simulink model "ATRIAS_vnmc"  (R2015a)
settings: Solver=ode45  StartTime=0.0  StopTime=60  FixedStep=1e-3  MinStep=1e-6  RelTol=1e-3  AbsTol=1e-4
values from neighbouring files (symbols this model uses):
  initial_boom_yaw = initial_boom_yaw + delta_yaw0    [run_model.m]
  max_floor_diff = cost_fun_opts.max_floor_diff    [opt_cmaes.m]    (also in run_model.m; set_all_params_simple.m = 0)
  noise_on_off = cost_fun_opts.noise_on_off    [opt_cmaes.m]    (also in run_model.m; set_all_params_simple.m = 0)
  noise_seed = cost_fun_opts.noise_seed    [opt_cmaes.m]    (also in run_model.m; set_all_params_simple.m = 1)
  noise_variance = cost_fun_opts.noise_variance    [opt_cmaes.m]    (also in run_model.m; set_all_params_simple.m = 0.000174532925199)
  SEA_swing_ctrl_on_off = cost_fun_opts.SEA_swing_ctrl_on_off    [opt_cmaes.m]    (also in run_model.m; set_all_params_simple.m = 0)
  sim_t = simout.twalk    [run_model.m]
  steady_dist = cost_fun_opts.steady_dist    [opt_cmaes.m]    (also in run_model.m; set_all_params_simple.m = 10)
  ts_anim = 0.0333    [run_model.m]
undefined symbols (not defined in the file or in its folder): A1_notch_f1, A2_notch_f1, A_lpf_dtau, A_lpf_velocity, B1_lpf_dtau, B1_lpf_velocity, B1_notch_f1, B2_lpf_dtau, B2_lpf_velocity, B2_notch_f1, b_hmotor, b_leg_spring, b_rotor, base_color_d, boom_color_d, boom_mount_to_center_diagonal, breakaway_friction, c, c_jointstop, com_height_offset, contactThr, coulomb_friction, CtrlPar_theta0, D12_S, D12_T, d_com, ddx_max, ddy_max, delta_phi_max, delta_phi_max_buffer, delta_phi_max_dropoff, delta_phi_min, des_forward_velocity, DS_width, dtau_des_max, dtheta0_vmc, dx0_vmc, dy_max, eref, fblink_color_d, fcut_acceleration, floor_color_d, floor_tile_width, floor_zero_height, FmaxBFSH, FmaxGLU, FmaxHAM, FmaxHFL, FmaxRF, FmaxVAS, FPCtrlPar, friction_linear_zone, g, gain_nodes_sea_torque, gamma_stance_thr, gamma_swing_thr, hip_height, HIP_MTR_MAX_CONT_TORQUE, HIP_MTR_MAX_TORQUE, hshaft_color_d ... (+236)
libraries: sm_lib x280, nesl_utility x174, simulink x114, simulink_extras x58, fl_lib x16, mblibv1 x2, dspswit3 x2
(part 1 of 23)
settings Model: CovSFcnEnable=off  ExtModeTrigDuration=100  TunableVars=CtrlPar_theta0,FPCtrlPar,LLCtrlPar,StCtrlPar,SwCtrlPar,TrCtrlPar,v_plateYaw,v_plateH,v_plateS,maxFloorDiff,noise_variance  TunableVarsStorageClass=Auto,Auto,Auto,Auto,Auto,Auto,Auto,Auto,Auto,Auto,Auto  TunableVarsTypeQualifier=,,,,,,,,,,  Creator=hgeyer  LastModifiedBy=smsong
settings SolverCC: ConsecutiveZCsStepRelTol=1e-8  MaxConsecutiveZCs=10  ZeroCrossControl=EnableAll  ZeroCrossAlgorithm=Adaptive
settings DataIOCC: LimitDataPoints=off  SaveFormat=StructureWithTime  SignalLoggingSaveFormat=ModelDataLogs  SaveOutput=off  SignalLogging=off  DSMLogging=off  SaveTime=off  ReturnWorkspaceOutputs=on
settings OptimizationCC: BooleanDataType=off  ExpressionDepthLimit=2147483647  InitFltsAndDblsToZero=on  EfficientMapNaN2IntZero=off  SimCompilerOptimization=on
settings DebuggingCC: SaveWithParameterizedLinksMsg=none  UnderspecifiedInitializationDetection=Classic  MergeDetectMultiDrivingBlocksExec=none  SignalResolutionControl=TryResolveAllWithWarning  MaxConsecutiveZCsMsg=none  MaskedZcDiagnostic=none  SolverPrmCheckMsg=warning  DiscreteInheritContinuousMsg=none  MultiTaskDSMMsg=warning  MultiTaskCondExecSysMsg=none  FcnCallInpInsideContextMsg=UseLocalSettings  StateNameClashWarn=warning
settings HardwareCC: TargetLongLongMode=on  TargetIntDivRoundTo=Zero  TargetEndianess=LittleEndian  TargetHWDeviceType=MATLAB Host  ProdEqTarget=off
settings RTWCC: SystemTargetFile=raccel.tlc  TemplateMakefile=raccel_default_tmf  RTWVerbose=off  RTWUseSimCustomCode=on
settings CodeAppCC: GenerateComments=off  MaxIdLength=128  MangleLength=10  SimulinkBlockComments=off
settings RaccelTargetCC: ERTMultiwordTypeDef=System defined  ERTMultiwordLength=256  GeneratePreprocessorConditionals=Disable all  ERTFirstTimeCompliant=off  MultiInstanceERTCode=off  ENABLE_SLEXEC_SSBRIDGE=0  RTWCAPIParams=off
settings SimscapeCC: ExplicitSolverDiagnosticOptions=none
settings SimMechanicsCC: VisOnUpdateDiagram=on  VisDuringSimulation=on  VisSampleTime=0.01  AutoFitVis=TIGHTFIT  LastVizWinPosition=[360 278 560 420]  CamPosition=[2.01156;0.662717;15.4496;]  CamTarget=[2.01156;0.662717;0;]  CamUpVector=[0;1;0;]  CamHeight=5.84419  VisBackgroundColor=[0.9;0.9;0.95;]  DefaultBodyColor=[1;0;0;]
settings DiagnosticsConfigSet: SimMechanicsUnconnectedFramePorts=none  SimMechanicsRigidlyBoundBlock=warning  SimMechanicsJointTargetOverSpecification=none

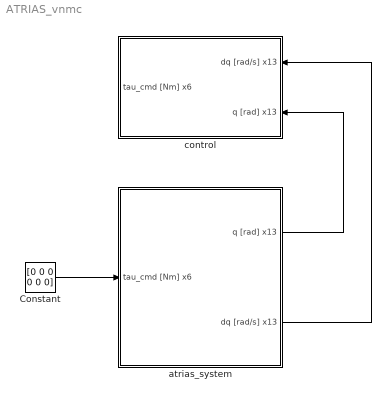
== system ATRIAS_vnmc ==
  Constant : Constant  Value=[0 0 0 0 0 0]
  atrias_system : Subsystem
  control : Subsystem
  wires:
  atrias_system/1(q [rad] x13) -> control/2(q [rad] x13)
  atrias_system/2(dq [rad/s] x13) -> control/1(dq [rad/s] x13)
  Constant/1 -> atrias_system/1(tau_cmd [Nm] x6)

== system ATRIAS_vnmc/atrias_system ==
  note: ATRIAS System
  note: Continuous Signal
  note: Encoders
  note: Continuous Signal
  note: Discrete Signal
  note: Continuous Signal
  tau_cmd [Nm] x6 : Inport
  ATRIAS Mechanical System Layer : Subsystem
  Demux : Demux  Outputs=6
  "Discretize Sensors, Add Noise" : Subsystem
  Ground Contact : Subsystem
  Mux1 : Mux  Inputs=13
  Mux2 : Mux  Inputs=13
  Mux3 : Mux  Inputs=2
  Mux4 : Mux  Inputs=13
  Mux5 : Mux
  Selector3 : Selector  InputPortWidth=6  Indices=[3 6]
  Selector8 : Selector  InputPortWidth=6  Indices=[1 2 5 3 4 6]
  Selector9 : Selector  InputPortWidth=6  Indices=[1 2 4 5]
  Simulation Lateral Motor Direction : Gain  Gain=-1
  Simulation Sagittal Motor Direction : Gain  Gain=-1
  Terminator : Terminator
  Terminator1 : Terminator
  Terminator2 : Terminator
  q [rad] x13 : Outport
  dq [rad/s] x13 : Outport  Port=2
  tag scope: L_rotor_stiction_back=global, L_rotor_stiction_front=global, R_rotor_stiction_back=global, R_rotor_stiction_front=global, ddq10=global, ddq11=global, ddq12=global, ddq13=global, ddq1=global, ddq2=global, ddq3=global, ddq4=global, ddq5=global, ddq6=global, ddq7=global, ddq8=global, ddq9=global, dq10=global, dq11=global, dq12=global, dq13=global, dq1=global, dq2=global, dq3=global, dq4=global, dq5=global, dq6=global, dq7=global, dq8=global, dq9=global, q10=global, q11=global, q12=global, q13=global, q1=global, q2=global, q3=global, q4=global, q5=global, q6=global, q7=global, q8=global, q9=global
  wires:
  Demux/1 -> ATRIAS Mechanical System Layer/1(R Back Motor [Nm])
  Demux/2 -> ATRIAS Mechanical System Layer/2(R Front Motor [Nm])
  Demux/3 -> ATRIAS Mechanical System Layer/3(R Lat Motor [Nm])
  Demux/4 -> ATRIAS Mechanical System Layer/4(L Back Motor [Nm])
  Demux/5 -> ATRIAS Mechanical System Layer/5(L Front Motor [Nm])
  Demux/6 -> ATRIAS Mechanical System Layer/6(L Lat Motor [Nm])
  tau_cmd [Nm] x6/1 -> Selector3/1, Selector9/1
  Selector3/1 -> Simulation Lateral Motor Direction/1  "lateral"
  Mux3/1 -> Selector8/1
  Simulation Sagittal Motor Direction/1 -> Mux3/1
  Selector9/1 -> Simulation Sagittal Motor Direction/1  "sagittal"
  Selector8/1 -> Demux/1
  Mux1/1 -> "Discretize Sensors, Add Noise"/1(q [rad] x13)
  [q1] -> Mux1/1
  [q2] -> Mux1/2
  [q4] -> Mux1/4
  [q3] -> Mux1/3
  [q5] -> Mux1/5
  [q6] -> Mux1/6
  [q7] -> Mux1/7
  [q8] -> Mux1/8
  [q9] -> Mux1/9
  [q10] -> Mux1/10
  [q11] -> Mux1/11
  [q12] -> Mux1/12
  [q13] -> Mux1/13
  "Discretize Sensors, Add Noise"/1(q_discrete [rad] x13) -> q [rad] x13/1
  "Discretize Sensors, Add Noise"/2(dq_discrete [rad/s] x13) -> dq [rad/s] x13/1
  ATRIAS Mechanical System Layer/1(R Back Joint [rad]) -> [q1]
  ATRIAS Mechanical System Layer/2(R Back Gear [rad]) -> [q2]
  ATRIAS Mechanical System Layer/3(R Front Joint [rad]) -> [q3]
  ATRIAS Mechanical System Layer/4(R Front Gear [rad]) -> [q4]
  ATRIAS Mechanical System Layer/5(L Back Joint [rad]) -> [q5]
  ATRIAS Mechanical System Layer/6(L Back Gear [rad]) -> [q6]
  ATRIAS Mechanical System Layer/7(L Front Joint [rad]) -> [q7]
  ATRIAS Mechanical System Layer/8(L Front Gear [rad]) -> [q8]
  ATRIAS Mechanical System Layer/9(R Lateral [rad]) -> [q9]
  ATRIAS Mechanical System Layer/10(L Lateral [rad]) -> [q10]
  ATRIAS Mechanical System Layer/11(Boom Roll [rad]) -> [q11]
  ATRIAS Mechanical System Layer/12(Boom Yaw [rad]) -> [q12]
  ATRIAS Mechanical System Layer/13(Boom Pitch [rad]) -> [q13]
  ATRIAS Mechanical System Layer/14(R Back Joint Velocity [rad/s]) -> [dq1]
  ATRIAS Mechanical System Layer/15(R Back Gear Velocity [rad/s]) -> [dq2]
  ATRIAS Mechanical System Layer/16(R Front Joint Velocity [rad/s]) -> [dq3]
  ATRIAS Mechanical System Layer/17(R Front Gear Velocity [rad/s]) -> [dq4]
  ATRIAS Mechanical System Layer/18(L Back Joint Velocity [rad/s]) -> [dq5]
  ATRIAS Mechanical System Layer/19(L Back Gear Velocity [rad/s]) -> [dq6]
  ATRIAS Mechanical System Layer/20(L Front Joint Velocity [rad/s]) -> [dq7]
  ATRIAS Mechanical System Layer/21(L Front Gear Velocity [rad/s]) -> [dq8]
  ATRIAS Mechanical System Layer/22(R Lateral Velocity [rad]) -> [dq9]
  ATRIAS Mechanical System Layer/23(L Lateral Velocity [rad/s]) -> [dq10]
  ATRIAS Mechanical System Layer/24(Boom Roll Velocity [rad/s]) -> [dq11]
  ATRIAS Mechanical System Layer/25(Boom Yaw Velocity [rad/s]) -> [dq12]
  ATRIAS Mechanical System Layer/26(Boom Pitch Velocity [rad/s]) -> [dq13]
  Mux2/1 -> Terminator/1
  [dq1] -> Mux2/1
  [dq2] -> Mux2/2
  [dq4] -> Mux2/4
  [dq3] -> Mux2/3
  [dq5] -> Mux2/5
  [dq6] -> Mux2/6
  [dq7] -> Mux2/7
  [dq8] -> Mux2/8
  [dq9] -> Mux2/9
  [dq10] -> Mux2/10
  [dq11] -> Mux2/11
  [dq12] -> Mux2/12
  [dq13] -> Mux2/13
  Simulation Lateral Motor Direction/1 -> Mux3/2
  ATRIAS Mechanical System Layer/27(R Back Joint Acceleration [rad/s^2]) -> [ddq1]
  ATRIAS Mechanical System Layer/28(R Back Gear Acceleration [rad/s^2]) -> [ddq2]
  ATRIAS Mechanical System Layer/29(R Front Joint Acceleration [rad/s^2]) -> [ddq3]
  ATRIAS Mechanical System Layer/30(R Front Gear Acceleration [rad/s^2]) -> [ddq4]
  ATRIAS Mechanical System Layer/31(L Back Joint Acceleration [rad/s^2]) -> [ddq5]
  ATRIAS Mechanical System Layer/32(L Back Gear Acceleration [rad/s^2]) -> [ddq6]
  ATRIAS Mechanical System Layer/33(L Front Joint Acceleration [rad/s^2]) -> [ddq7]
  ATRIAS Mechanical System Layer/34(L Front Gear Acceleration [rad/s^2]) -> [ddq8]
  ATRIAS Mechanical System Layer/35(R Lateral Acceleration [rad/s^2]) -> [ddq9]
  ATRIAS Mechanical System Layer/36(L Lateral Acceleration [rad/s^2]) -> [ddq10]
  ATRIAS Mechanical System Layer/37(Boom Roll Acceleration [rad/s^2]) -> [ddq11]
  ATRIAS Mechanical System Layer/38(Boom Yaw Acceleration [rad/s^2]) -> [ddq12]
  ATRIAS Mechanical System Layer/39(Boom Pitch Acceleration [rad/s^2]) -> [ddq13]
  Mux4/1 -> Terminator1/1
  [ddq1] -> Mux4/1
  [ddq2] -> Mux4/2
  [ddq4] -> Mux4/4
  [ddq3] -> Mux4/3
  [ddq5] -> Mux4/5
  [ddq6] -> Mux4/6
  [ddq7] -> Mux4/7
  [ddq8] -> Mux4/8
  [ddq9] -> Mux4/9
  [ddq10] -> Mux4/10
  [ddq11] -> Mux4/11
  [ddq12] -> Mux4/12
  [ddq13] -> Mux4/13
  ATRIAS Mechanical System Layer/40(R Back Rotor Stiction [Nm]) -> [R_rotor_stiction_back]
  ATRIAS Mechanical System Layer/41(R Front Rotor Stiction [Nm]) -> [R_rotor_stiction_front]
  ATRIAS Mechanical System Layer/42(L Back Rotor Stiction [Nm]) -> [L_rotor_stiction_back]
  ATRIAS Mechanical System Layer/43(L Front Rotor Stiction [Nm]) -> [L_rotor_stiction_front]
  [R_rotor_stiction_back] -> Mux5/1
  [R_rotor_stiction_front] -> Mux5/2
  [L_rotor_stiction_back] -> Mux5/3
  [L_rotor_stiction_front] -> Mux5/4
  Mux5/1 -> Terminator2/1
  connections:
  ATRIAS Mechanical System Layer/RConn1 -- Ground Contact/RConn1
  ATRIAS Mechanical System Layer/LConn1 -- Ground Contact/LConn1

== system ATRIAS_vnmc/control ==
  note: Robot-NMM Interface
  note: Neuromuscular Model
  note: Data
  note: Lateral Motors
  note: Avoid Limits
  note: SEA Control
  note: Virtual Model Control
  note: Switch
  dq [rad/s] x13 : Inport
  q [rad] x13 : Inport  Port=2
  Add Limit Avoidance PD Torques : Subsystem
  Constant1 : Constant  Value=[1,1,1,1]
  Constant2 : Constant  Value=SEA_swing_ctrl_on_off
  Data Type Conversion : DataTypeConversion  OutDataTypeStr=boolean
  Data Type Conversion1 : DataTypeConversion  OutDataTypeStr=boolean
  Demux : Demux  Outputs=6
  Demux1 : Demux  Outputs=6
  Demux2 : Demux
  Demux3 : Demux
  Export Results : Subsystem
  Import Control Parameters : Subsystem
  Lateral Motor Control : Subsystem
  Monitor Simulation : Subsystem
  Mux : Mux  Inputs=6
  Mux1 : Mux  Inputs=2
  Mux2 : Mux  Inputs=6
  Mux3 : Mux  Inputs=2
  Mux4 : Mux  Inputs=6
  Mux5 : Mux  Inputs=2
  Mux6 : Mux
  Mux7 : Mux
  Mux8 : Mux
  Plot Signals : Subsystem
  Robot-to-NMM Interface : Subsystem
  SEA Ctrl : Subsystem
  Switch : Switch  Criteria=u2 ~= 0
  Switch2 : Switch  Criteria=u2 ~= 0
  Turn on NMM : Subsystem
  Virtual Model Control : Subsystem  SystemSampleTime=sample_time
  Virtual Neuromuscular Control : Subsystem  SystemSampleTime=sample_time
  tau_cmd [Nm] x6 : Outport
  tag scope: LFootCnt=global, LLLoad=global, LLat_cmd_trq=global, LLat_ctrl_trq=global, LLength=global, Lalpha=global, LdLength=global, Ldalpha=global, Ldgamma=global, Lgamma=global, Lphi12=global, Lphi23=global, Lshin_cmd_trq=global, Lshin_ctrl_trq=global, Lshin_ctrl_trq_NMM=global, Lshin_ctrl_trq_VMC=global, Lshin_des_trq=global, LtauB=global, LtauF=global, Lthigh_cmd_trq=global, Lthigh_ctrl_trq=global, Lthigh_ctrl_trq_NMM=global, Lthigh_ctrl_trq_VMC=global, Lthigh_des_trq=global, RFootCnt=global, RLLoad=global, RLat_cmd_trq=global, RLat_ctrl_trq=global, RLength=global, Ralpha=global, RdLength=global, Rdalpha=global, Rdgamma=global, Rgamma=global, Rphi12=global, Rphi23=global, Rshin_cmd_trq=global, Rshin_ctrl_trq=global, Rshin_ctrl_trq_NMM=global, Rshin_ctrl_trq_VMC=global, Rshin_des_trq=global, RtauB=global, RtauF=global, Rthigh_cmd_trq=global, Rthigh_ctrl_trq=global, Rthigh_ctrl_trq_NMM=global, Rthigh_ctrl_trq_VMC=global, Rthigh_des_trq=global, dLshin_des_trq=global, dLthigh_des_trq=global, dRshin_des_trq=global, dRthigh_des_trq=global, dq=global, k_L=global, k_R=global, q=global
  wires:
  [q] -> SEA Ctrl/4(q)
  [dq] -> SEA Ctrl/5(dq)
  Mux5/1 -> Mux1/2
  Mux3/1 -> Mux1/1
  [RFootCnt] -> Mux3/2, Mux3/1
  [LFootCnt] -> Mux5/1, Mux5/2
  Mux1/1 -> Data Type Conversion/1
  Demux/1 -> [Rshin_cmd_trq]
  Demux/2 -> [Rthigh_cmd_trq]
  Demux/3 -> [RLat_cmd_trq]
  Demux/4 -> [Lshin_cmd_trq]
  Demux/5 -> [Lthigh_cmd_trq]
  Demux/6 -> [LLat_cmd_trq]
  [Rshin_ctrl_trq] -> Mux/1
  [Rthigh_ctrl_trq] -> Mux/2
  [RLat_ctrl_trq] -> Mux/3
  [Lshin_ctrl_trq] -> Mux/4
  [Lthigh_ctrl_trq] -> Mux/5
  [LLat_ctrl_trq] -> Mux/6
  Mux/1 -> Add Limit Avoidance PD Torques/1(tau_des [Nm] x6)
  [Rshin_cmd_trq] -> Mux2/1
  [Rthigh_cmd_trq] -> Mux2/2
  [RLat_cmd_trq] -> Mux2/3
  [Lshin_cmd_trq] -> Mux2/4
  [Lthigh_cmd_trq] -> Mux2/5
  [LLat_cmd_trq] -> Mux2/6
  SEA Ctrl/1(tau_cmd [Nm] x6) -> Demux/1
  dq [rad/s] x13/1 -> [dq]
  q [rad] x13/1 -> [q]
  Mux2/1 -> tau_cmd [Nm] x6/1
  [Rshin_des_trq] -> Mux4/1
  [Rthigh_des_trq] -> Mux4/2
  [Lshin_des_trq] -> Mux4/4
  [Lthigh_des_trq] -> Mux4/5
  Demux1/1 -> [Rshin_des_trq]
  Demux1/2 -> [Rthigh_des_trq]
  Demux1/4 -> [Lshin_des_trq]
  Demux1/5 -> [Lthigh_des_trq]
  Demux1/3 -> Mux4/3  "no change"
  Demux1/6 -> Mux4/6  "no change"
  Mux4/1 -> SEA Ctrl/1(Desired Torque [Nm] x6)
  Add Limit Avoidance PD Torques/1(tau_des w/PD [Nm] x6) -> Demux1/1
  Mux6/1 -> SEA Ctrl/2(Desired SEA Torque Velocity [Nm] x4)
  Demux2/1 -> [dRshin_des_trq]
  Demux2/3 -> [dLshin_des_trq]
  Demux2/4 -> [dLthigh_des_trq]
  Demux2/2 -> [dRthigh_des_trq]
  [dLshin_des_trq] -> Mux6/3
  [dLthigh_des_trq] -> Mux6/4
  [dRthigh_des_trq] -> Mux6/2
  [dRshin_des_trq] -> Mux6/1
  Add Limit Avoidance PD Torques/2(d/dt[tau_des w/PD] [Nm/s] x4) -> Demux2/1
  Constant1/1 -> Data Type Conversion1/1
  Data Type Conversion1/1 -> Switch/1
  Data Type Conversion/1 -> Switch/3
  Constant2/1 -> Switch/2
  Switch/1 -> SEA Ctrl/3(Enable SEA Control [1/0] x4)
  [q] -> Robot-to-NMM Interface/1(q_discrete [rad] x13)
  [dq] -> Robot-to-NMM Interface/2(dq_discrete [rad/2] x13)
  Robot-to-NMM Interface/6(L Leg Load [bw]) -> [LLLoad]
  Robot-to-NMM Interface/5(R Leg Load [bw]) -> [RLLoad]
  Robot-to-NMM Interface/10(L Alpha [rad]) -> [Lalpha]
  Robot-to-NMM Interface/9(R Alpha [rad]) -> [Ralpha]
  Robot-to-NMM Interface/14(L Leg Length [m]) -> [LLength]
  Robot-to-NMM Interface/13(R Leg Length [m]) -> [RLength]
  Robot-to-NMM Interface/7(R Contact [0/1]) -> [RFootCnt]
  Robot-to-NMM Interface/8(L Contact [0/1]) -> [LFootCnt]
  Robot-to-NMM Interface/4(L_tau_front_meas [Nm]) -> [LtauF]
  Robot-to-NMM Interface/3(L_tau_back_meas [Nm]) -> [LtauB]
  Robot-to-NMM Interface/2(R_tau_front_meas [Nm]) -> [RtauF]
  Robot-to-NMM Interface/1(R_tau_back_meas [Nm]) -> [RtauB]
  Robot-to-NMM Interface/17(R virtual knee angle [rad]) -> [Rphi12]
  Robot-to-NMM Interface/18(R virtual hip angle [rad]) -> [Rphi23]
  Robot-to-NMM Interface/19(L virtual knee angle [rad]) -> [Lphi12]
  Robot-to-NMM Interface/20(L virtual hip angle [rad]) -> [Lphi23]
  Robot-to-NMM Interface/22(L Jacobian Constant (k)) -> [k_L]
  Robot-to-NMM Interface/21(R Jacobian Constant (k)) -> [k_R]
  Robot-to-NMM Interface/11(R dAlpha [rad/s]) -> [Rdalpha]
  Robot-to-NMM Interface/12(L dAlpha [rad/s]) -> [Ldalpha]
  Robot-to-NMM Interface/23(Rgamma [rad]) -> [Rgamma]
  Robot-to-NMM Interface/24(Lgamma [rad]) -> [Lgamma]
  Robot-to-NMM Interface/25(Rdgamma [rad]) -> [Rdgamma]
  Robot-to-NMM Interface/26(Ldgamma [rad]) -> [Ldgamma]
  Robot-to-NMM Interface/15(R Leg Length Velocity [m/s]) -> [RdLength]
  Robot-to-NMM Interface/16(L Leg Length Velocity [m/s]) -> [LdLength]
  Virtual Model Control/1(Rtau_B_des [Nm]) -> [Rshin_ctrl_trq_VMC]
  Virtual Model Control/2(Rtau_F_des [Nm]) -> [Rthigh_ctrl_trq_VMC]
  Virtual Model Control/3(Ltau_B_des [Nm]) -> [Lshin_ctrl_trq_VMC]
  Virtual Model Control/4(Ltau_F_des [Nm]) -> [Lthigh_ctrl_trq_VMC]
  Virtual Neuromuscular Control/1(RtauB_des [Nm]) -> [Rshin_ctrl_trq_NMM]
  Virtual Neuromuscular Control/2(RtauF_des [Nm]) -> [Rthigh_ctrl_trq_NMM]
  Virtual Neuromuscular Control/3(LtauB_des [Nm]) -> [Lshin_ctrl_trq_NMM]
  Virtual Neuromuscular Control/4(LtauF_des [Nm]) -> [Lthigh_ctrl_trq_NMM]
  Turn on NMM/1(Turn on NMM) -> Switch2/2
  [Rshin_ctrl_trq_NMM] -> Mux7/1
  [Rthigh_ctrl_trq_NMM] -> Mux7/2
  [Lshin_ctrl_trq_NMM] -> Mux7/3
  [Lthigh_ctrl_trq_NMM] -> Mux7/4
  Mux7/1 -> Switch2/1
  [Rshin_ctrl_trq_VMC] -> Mux8/1
  [Rthigh_ctrl_trq_VMC] -> Mux8/2
  [Lshin_ctrl_trq_VMC] -> Mux8/3
  [Lthigh_ctrl_trq_VMC] -> Mux8/4
  Mux8/1 -> Switch2/3
  Switch2/1 -> Demux3/1
  Demux3/4 -> [Lthigh_ctrl_trq]
  Demux3/3 -> [Lshin_ctrl_trq]
  Demux3/2 -> [Rthigh_ctrl_trq]
  Demux3/1 -> [Rshin_ctrl_trq]
  Lateral Motor Control/2(tau_lateral_L) -> [LLat_ctrl_trq]
  Lateral Motor Control/1(tau_lateral_R) -> [RLat_ctrl_trq]

== system ATRIAS_vnmc/atrias_system/ATRIAS Mechanical System Layer ==
  R Back Motor [Nm] : Inport
  R Front Motor [Nm] : Inport  Port=2
  R Lat Motor [Nm] : Inport  Port=3
  L Back Motor [Nm] : Inport  Port=4
  L Front Motor [Nm] : Inport  Port=5
  L Lat Motor [Nm] : Inport  Port=6
  Boom : Subsystem
      mask Display: image(imread('../0_images/images/boom.png'));
  Boom Base : Subsystem
      mask Display: image(imread('../0_images/images/boom_base.png'));
  Floor Frame1 : sm_lib/Frames and Transforms/Rigid Transform  TranslationMethod=Cartesian  TranslationLengthUnit=m  TranslationStandardAxis=+Z  TranslationStandardOffset=0  TranslationCartesianOffset=[0 -floor_zero_height 0]  TranslationROffset=0  TranslationROffsetUnits=m  TranslationZOffset=0  TranslationZOffsetUnits=m  TranslationThetaOffset=0  TranslationThetaOffsetUnits=deg  RotationMethod=AlignedAxes  RotationAngleUnits=deg  RotationStandardAxis=+Z  RotationAngle=0  RotationArbitraryAxis=[0 0 1]  FollAlignAxisA=+Z  BaseAlignAxisA=+Y  FollAlignAxisB=+X  BaseAlignAxisB=+X  RotationMatrix=[1 0 0; 0 1 0; 0 0 1]  BlockFunction=simmechanics.library.frames_transforms.rigid_transform
  Floor Visualization : Subsystem
  Ground : Subsystem
  L Hip Shaft : Subsystem
      mask Display: image(flipdim(imread('../0_images/images/hipshaft.JPG'),2));
  L Leg : Subsystem
      mask Display: image(imread('../0_images/images/leg.JPG'));
  L Virtual Leg Visualization : Subsystem  Commented=on
  L Virtual Leg Visualization1 : Subsystem
  Lalpha_tgt Visualization : Subsystem  Commented=on
  Left Hip Roll Joint : Subsystem
  Pitch Joint : Subsystem
  R Hip Shaft : Subsystem
      mask Display: image(imread('../0_images/images/hipshaft.JPG'));
  R Leg : Subsystem
      mask Display: image(imread('../0_images/images/leg.JPG'));
  R Virtual Leg Visualization : Subsystem  Commented=on
  R Virtual Leg Visualization1 : Subsystem
  Ralpha_tgt Visualization : Subsystem  Commented=on
  Right Hip Roll Joint : Subsystem
  Torso : Subsystem
      mask Display: image(imread('../0_images/images/torso.png'));
  Winch : Subsystem
  Yaw Joint : Subsystem
  Yaw Shaft : Subsystem
      mask Display: image(imread('../0_images/images/boom_yaw_shaft.png'));
  gamma min/max visualization : Subsystem
  gamma min/max visualization1 : Subsystem
  R Ground Contact : PMIOPort  Port=1  Side=Right
  L Ground Contact : PMIOPort  Port=2  Side=Left
  R Back Joint [rad] : Outport
  R Back Gear [rad] : Outport  Port=2
  R Front Joint [rad] : Outport  Port=3
  R Front Gear [rad] : Outport  Port=4
  L Back Joint [rad] : Outport  Port=5
  L Back Gear [rad] : Outport  Port=6
  L Front Joint [rad] : Outport  Port=7
  L Front Gear [rad] : Outport  Port=8
  R Lateral [rad] : Outport  Port=9
  L Lateral [rad] : Outport  Port=10
  Boom Roll [rad] : Outport  Port=11
  Boom Yaw [rad] : Outport  Port=12
  Boom Pitch [rad] : Outport  Port=13
  R Back Joint Velocity [rad/s] : Outport  Port=14
  R Back Gear Velocity [rad/s] : Outport  Port=15
  R Front Joint Velocity [rad/s] : Outport  Port=16
  R Front Gear Velocity [rad/s] : Outport  Port=17
  L Back Joint Velocity [rad/s] : Outport  Port=18
  L Back Gear Velocity [rad/s] : Outport  Port=19
  L Front Joint Velocity [rad/s] : Outport  Port=20
  L Front Gear Velocity [rad/s] : Outport  Port=21
  R Lateral Velocity [rad] : Outport  Port=22
  L Lateral Velocity [rad/s] : Outport  Port=23
  Boom Roll Velocity [rad/s] : Outport  Port=24
  Boom Yaw Velocity [rad/s] : Outport  Port=25
  Boom Pitch Velocity [rad/s] : Outport  Port=26
  R Back Joint Acceleration [rad/s^2] : Outport  Port=27
  R Back Gear Acceleration [rad/s^2] : Outport  Port=28
  R Front Joint Acceleration [rad/s^2] : Outport  Port=29
  R Front Gear Acceleration [rad/s^2] : Outport  Port=30
  L Back Joint Acceleration [rad/s^2] : Outport  Port=31
  L Back Gear Acceleration [rad/s^2] : Outport  Port=32
  L Front Joint Acceleration [rad/s^2] : Outport  Port=33
  L Front Gear Acceleration [rad/s^2] : Outport  Port=34
  R Lateral Acceleration [rad/s^2] : Outport  Port=35
  L Lateral Acceleration [rad/s^2] : Outport  Port=36
  Boom Roll Acceleration [rad/s^2] : Outport  Port=37
  Boom Yaw Acceleration [rad/s^2] : Outport  Port=38
  Boom Pitch Acceleration [rad/s^2] : Outport  Port=39
  R Back Rotor Stiction [Nm] : Outport  Port=40
  R Front Rotor Stiction [Nm] : Outport  Port=41
  L Back Rotor Stiction [Nm] : Outport  Port=42
  L Front Rotor Stiction [Nm] : Outport  Port=43
  wires:
  L Leg/1(Shin Joint [rad]) -> L Back Joint [rad]/1
  R Back Motor [Nm]/1 -> R Leg/1(Shin Motor [Nm])
  L Back Motor [Nm]/1 -> L Leg/1(Shin Motor [Nm])
  Right Hip Roll Joint/1(Hip Roll [rad]) -> R Lateral [rad]/1
  L Leg/3(Thigh Joint [rad]) -> L Front Joint [rad]/1
  Winch/1(Boom Roll [rad]) -> Boom Roll [rad]/1
  Left Hip Roll Joint/1(Hip Roll [rad]) -> L Lateral [rad]/1
  L Leg/4(Thigh Gear [rad]) -> L Front Gear [rad]/1
  R Leg/1(Shin Joint [rad]) -> R Back Joint [rad]/1
  R Leg/2(Shin Gear [rad]) -> R Back Gear [rad]/1
  L Leg/2(Shin Gear [rad]) -> L Back Gear [rad]/1
  R Leg/4(Thigh Gear [rad]) -> R Front Gear [rad]/1
  L Front Motor [Nm]/1 -> L Leg/2("Thigh Motor [Nm]  ")
  R Lat Motor [Nm]/1 -> Right Hip Roll Joint/1(Hip Motor [Nm])
  R Front Motor [Nm]/1 -> R Leg/2("Thigh Motor [Nm]  ")
  L Lat Motor [Nm]/1 -> Left Hip Roll Joint/1(Hip Motor [Nm])
  R Leg/3(Thigh Joint [rad]) -> R Front Joint [rad]/1
  Pitch Joint/1(Pitch [rad]) -> Boom Pitch [rad]/1
  Yaw Joint/1(Yaw [rad]) -> Boom Yaw [rad]/1
  R Leg/5(Shin Joint Velocity [rad/s]) -> R Back Joint Velocity [rad/s]/1
  R Leg/6(Shin Gear Velocity [rad/s]) -> R Back Gear Velocity [rad/s]/1
  R Leg/7(Thigh Joint Velocity [rad/s]) -> R Front Joint Velocity [rad/s]/1
  R Leg/8(Thigh Gear Velocity [rad/s]) -> R Front Gear Velocity [rad/s]/1
  L Leg/5(Shin Joint Velocity [rad/s]) -> L Back Joint Velocity [rad/s]/1
  L Leg/6(Shin Gear Velocity [rad/s]) -> L Back Gear Velocity [rad/s]/1
  L Leg/7(Thigh Joint Velocity [rad/s]) -> L Front Joint Velocity [rad/s]/1
  L Leg/8(Thigh Gear Velocity [rad/s]) -> L Front Gear Velocity [rad/s]/1
  Right Hip Roll Joint/2(Hip Roll Velocity [rad/s]) -> R Lateral Velocity [rad]/1
  Left Hip Roll Joint/2(Hip Roll Velocity [rad/s]) -> L Lateral Velocity [rad/s]/1
  Winch/2(Boom Roll Velocity [rad/s]) -> Boom Roll Velocity [rad/s]/1
  Yaw Joint/2(Yaw Velocity [rad/s]) -> Boom Yaw Velocity [rad/s]/1
  Pitch Joint/2(Pitch Velocity [rad/s]) -> Boom Pitch Velocity [rad/s]/1
  R Leg/9(Shin Joint Acceleration [rad/s^2]) -> R Back Joint Acceleration [rad/s^2]/1
  R Leg/10(Shin Gear Acceleration [rad/s^2]) -> R Back Gear Acceleration [rad/s^2]/1
  R Leg/11(Thigh Joint Acceleration [rad/s^2]) -> R Front Joint Acceleration [rad/s^2]/1
  R Leg/12(Thigh Gear Acceleration [rad/s^2]) -> R Front Gear Acceleration [rad/s^2]/1
  L Leg/9(Shin Joint Acceleration [rad/s^2]) -> L Back Joint Acceleration [rad/s^2]/1
  L Leg/10(Shin Gear Acceleration [rad/s^2]) -> L Back Gear Acceleration [rad/s^2]/1
  L Leg/11(Thigh Joint Acceleration [rad/s^2]) -> L Front Joint Acceleration [rad/s^2]/1
  L Leg/12(Thigh Gear Acceleration [rad/s^2]) -> L Front Gear Acceleration [rad/s^2]/1
  Left Hip Roll Joint/3(Hip Roll Acceleration [rad/s^2]) -> L Lateral Acceleration [rad/s^2]/1
  Right Hip Roll Joint/3(Hip Roll Acceleration [rad/s^2]) -> R Lateral Acceleration [rad/s^2]/1
  Winch/3(Boom Roll Acceleration [rad/s^2]) -> Boom Roll Acceleration [rad/s^2]/1
  Yaw Joint/3(Yaw Acceleration [rad/s^2]) -> Boom Yaw Acceleration [rad/s^2]/1
  Pitch Joint/3(Pitch Acceleration[rad/s^2]) -> Boom Pitch Acceleration [rad/s^2]/1
  R Leg/13(Shin Rotor Stiction [Nm]) -> R Back Rotor Stiction [Nm]/1
  R Leg/14(Thigh Rotor Stiction [Nm]) -> R Front Rotor Stiction [Nm]/1
  L Leg/13(Shin Rotor Stiction [Nm]) -> L Back Rotor Stiction [Nm]/1
  L Leg/14(Thigh Rotor Stiction [Nm]) -> L Front Rotor Stiction [Nm]/1
  connections:
  Torso/LConn1 -- Left Hip Roll Joint/RConn1
  Right Hip Roll Joint/RConn1 -- R Hip Shaft/RConn1
  Winch/RConn2 -- Yaw Shaft/RConn1
  Left Hip Roll Joint/LConn1 -- L Hip Shaft/LConn1
  R Ground Contact/RConn1 -- R Leg/LConn1
  R Virtual Leg Visualization/RConn1 -- R Leg/RConn1 -- gamma min/max visualization1/RConn1 -- R Virtual Leg Visualization1/RConn1 -- Ralpha_tgt Visualization/RConn1 -- R Hip Shaft/LConn1
  Torso/LConn2 -- Right Hip Roll Joint/LConn1
  L Virtual Leg Visualization/RConn1 -- gamma min/max visualization/RConn1 -- L Virtual Leg Visualization1/RConn1 -- L Leg/LConn1 -- L Hip Shaft/RConn1 -- Lalpha_tgt Visualization/RConn1
  L Ground Contact/RConn1 -- L Leg/RConn1
  Pitch Joint/LConn1 -- Torso/RConn1
  Ground/RConn1 -- Boom Base/LConn1 -- Floor Frame1/LConn1
  Boom/LConn1 -- Winch/RConn1
  Yaw Shaft/LConn1 -- Yaw Joint/RConn1
  Yaw Joint/LConn1 -- Boom Base/RConn1
  Pitch Joint/RConn1 -- Boom/RConn1
  Floor Frame1/RConn1 -- Floor Visualization/LConn1

== system ATRIAS_vnmc/atrias_system/Discretize Sensors, Add Noise ==
  q [rad] x13 : Inport
  Constant : Constant  Value=noise_on_off
  "Low Pass Discrete Derivative f(sample_time, A_lpf_velocity, B1_lpf_velocity, B2_lpf_velocity)" : Subsystem
  "Random Number f(noise_seed, sample_time) variance = 1" : RandomNumber  Seed=noise_seed  SampleTime=sample_time
  Sum : Sum  Inputs=|++
  Zero-Order Hold f(sample_time) : ZeroOrderHold  SampleTime=sample_time
  "scale by noise_variance, saturate by [-3*noise_variance,3*noise_variance]" : Subsystem  TreatAsAtomicUnit=on
  q_discrete [rad] x13 : Outport
  dq_discrete [rad/s] x13 : Outport  Port=2
  wires:
  Sum/1 -> q_discrete [rad] x13/1, "Low Pass Discrete Derivative f(sample_time, A_lpf_velocity, B1_lpf_velocity, B2_lpf_velocity)"/1(q)
  "Random Number f(noise_seed, sample_time) variance = 1"/1 -> "scale by noise_variance, saturate by [-3*noise_variance,3*noise_variance]"/1(Variance = 1)
  q [rad] x13/1 -> Zero-Order Hold f(sample_time)/1
  "scale by noise_variance, saturate by [-3*noise_variance,3*noise_variance]"/1(Variance = noise_variance) -> Sum/2
  Zero-Order Hold f(sample_time)/1 -> Sum/1
  "Low Pass Discrete Derivative f(sample_time, A_lpf_velocity, B1_lpf_velocity, B2_lpf_velocity)"/1(dq) -> dq_discrete [rad/s] x13/1
  Constant/1 -> "scale by noise_variance, saturate by [-3*noise_variance,3*noise_variance]"/Enable

== system ATRIAS_vnmc/atrias_system/Ground Contact ==
  note: *********************************
      |
      |
      | Both ground contacts must start [yaw > 0],
      | due to the way yaw is calculated.
      |
      |
      |
      | *********************************
  L Contact : Subsystem
  R Contact : Subsystem
  roundTrack (LFoot) : Subsystem
  roundTrack (RFoot) : Subsystem
  L : PMIOPort  Port=1  Side=Left
  R : PMIOPort  Port=2  Side=Right
  tag scope: Env_LFoot=global, Env_RFoot=global, LHeelCont=global, LHeel_GRF=global, LxyzHeel=global, RHeelCont=global, RHeel_GRF=global, RxyzHeel=global
  wires:
  L Contact/2(GRF [N N N]) -> [LHeel_GRF]
  L Contact/3(xyzFoot) -> [LxyzHeel]
  L Contact/1(RBallCnt) -> [LHeelCont]
  [Env_LFoot] -> L Contact/1(Env)
  R Contact/2(GRF [N N N]) -> [RHeel_GRF]
  R Contact/3(xyzFoot) -> [RxyzHeel]
  R Contact/1(RBallCnt) -> [RHeelCont]
  [Env_RFoot] -> R Contact/1(Env)
  roundTrack (LFoot)/1(Env) -> [Env_LFoot]
  [LxyzHeel] -> roundTrack (LFoot)/1(Cnt)
  roundTrack (RFoot)/1(Env) -> [Env_RFoot]
  [RxyzHeel] -> roundTrack (RFoot)/1(Cnt)
  connections:
  R/RConn1 -- R Contact/LConn1
  L/RConn1 -- L Contact/LConn1

== system ATRIAS_vnmc/control/Add Limit Avoidance PD Torques ==
  tau_des [Nm] x6 : Inport
  Mux4 : Mux  Inputs=2
  Selector2 : Selector  InputPortWidth=6  Indices=[1 2 4 5]
  Selector3 : Selector  InputPortWidth=6  Indices=[3 6]
  Selector33 : Selector  InputPortWidth=6  Indices=[1 2 4 5]
  Selector8 : Selector  InputPortWidth=6  Indices=[1 2 5 3 4 6]
  Zero-Order Hold (1kHz)4 : ZeroOrderHold  SampleTime=sample_time
  dtau_des : Subsystem
  mechanical limit avoidance : Subsystem
  tau_des w/PD [Nm] x6 : Outport
  d/dt[tau_des w/PD] [Nm/s] x4 : Outport  Port=2
  wires:
  Selector33/1 -> dtau_des/1(x)
  dtau_des/1(dx/dt) -> d/dt[tau_des w/PD] [Nm/s] x4/1
  Zero-Order Hold (1kHz)4/1 -> Selector2/1, Selector3/1
  tau_des [Nm] x6/1 -> Zero-Order Hold (1kHz)4/1
  Selector8/1 -> tau_des w/PD [Nm] x6/1, Selector33/1
  Mux4/1 -> Selector8/1
  Selector3/1 -> Mux4/2
  Selector2/1 -> mechanical limit avoidance/1(tau_des [Nm]x4)
  mechanical limit avoidance/1(tau_des + pd [Nm]x4) -> Mux4/1

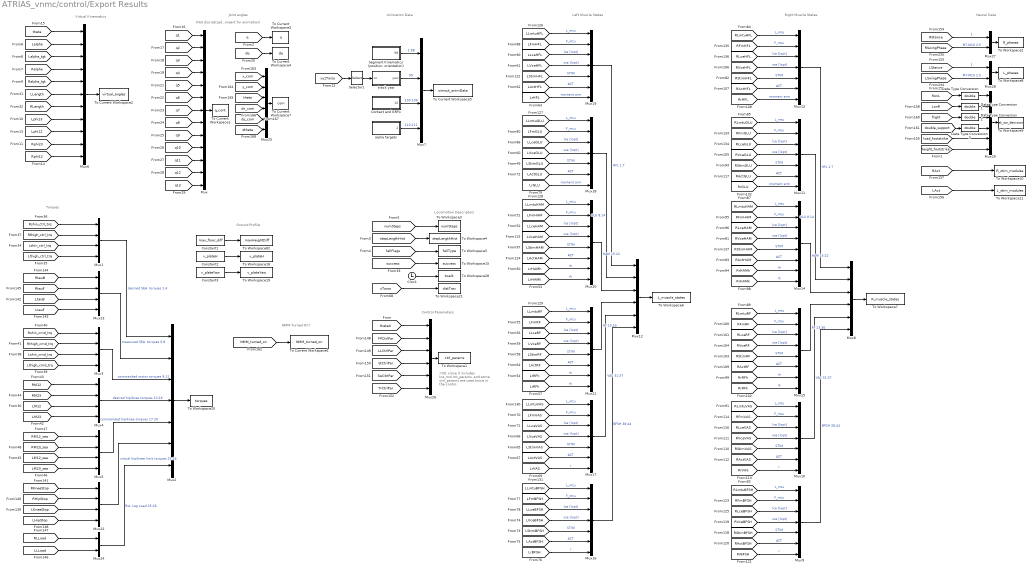
== system ATRIAS_vnmc/control/Export Results ==
  note: >50, since it includes
      | lce_msl.mt_params, and some
      | ctrl_params are used twice
      | in the contro
  note: (Not discretized...meant for animation)
  note: Animation Data
  note: Joint angles
  note: Virtual Kinematics
  note: Torques
  note: Right Muscle States
  note: Left Muscle States
  note: Locomotion Descriptors
  note: Ground Profile
  note: Neural Data
  note: Control Parameters
  note: NMM Turned On?
  Clock : Clock
  Constant1 : Constant  Value=max_floor_diff
  Constant2 : Constant  Value=v_plateH
  Constant3 : Constant  Value=v_plateYaw
  Contact and GRFs : Subsystem
  Data Type Conversion{,1..3} (4 alike) : DataTypeConversion  OutDataTypeStr=double
  Mux : Mux  Inputs=13
  Mux{1,3..5,7,22..23} (7 alike) : Mux
  Mux{2,9..11,13,16..19} (9 alike) : Mux  Inputs=7
  Mux{8,12,25..26,29} (5 alike) : Mux  Inputs=6
  Mux{14..15,20..21} (4 alike) : Mux  Inputs=8
  Mux24 : Mux  Inputs=2
  Mux27 : Mux  Inputs=2
  Mux28 : Mux  Inputs=2
  Mux6 : Mux  Inputs=11
  "Segment Kinematics (position, orientation)" : Subsystem
  Selector1 : Selector  InputPortWidth=3  Indices=[1 3]
  To Current Workspace1 : ToWorkspace  VariableName=q_cont  SaveFormat=Structure With Time  SampleTime=ts_anim
  To Current Workspace2 : ToWorkspace  VariableName=virtual_angles  SampleTime=ts_data
  To Current Workspace3 : ToWorkspace  VariableName=q  SampleTime=ts_data
  To Current Workspace4 : ToWorkspace  VariableName=dq  SampleTime=ts_data
  To Current Workspace5 : ToWorkspace  VariableName=simout_animData  SaveFormat=Structure With Time  SampleTime=ts_anim
  To Current Workspace6 : ToWorkspace  VariableName=NMM_turned_on  SampleTime=ts_data
  To Current Workspace7 : ToWorkspace  VariableName=com  SampleTime=ts_data
  To Workspace1 : ToWorkspace  VariableName=ctrl_params  SampleTime=-1
      settings: MaxDataPoints=1
  To Workspace10 : ToWorkspace  VariableName=R_stim_modules  SampleTime=ts_data
      settings: MaxDataPoints=Inf
  To Workspace11 : ToWorkspace  VariableName=L_stim_modules  SampleTime=ts_data
      settings: MaxDataPoints=Inf
  To Workspace15 : ToWorkspace  VariableName=success  SampleTime=-1
      settings: MaxDataPoints=1
  To Workspace18 : ToWorkspace  VariableName=v_plateH  SampleTime=-1
      settings: MaxDataPoints=1
  To Workspace19 : ToWorkspace  VariableName=v_plateYaw  SampleTime=-1
      settings: MaxDataPoints=1
  To Workspace2 : ToWorkspace  VariableName=R_phases  SampleTime=ts_data
      settings: MaxDataPoints=Inf
  To Workspace20 : ToWorkspace  VariableName=torques  SampleTime=ts_data
      settings: MaxDataPoints=Inf
  To Workspace21 : ToWorkspace  VariableName=distTrav  SampleTime=-1
      settings: MaxDataPoints=1
  To Workspace28 : ToWorkspace  VariableName=twalk  SampleTime=-1
      settings: MaxDataPoints=1
  To Workspace3 : ToWorkspace  VariableName=numSteps  SampleTime=-1
      settings: MaxDataPoints=1
  To Workspace4 : ToWorkspace  VariableName=stepLengthHist  SampleTime=-1
      settings: MaxDataPoints=1
  To Workspace5 : ToWorkspace  VariableName=fallType  SampleTime=-1
      settings: MaxDataPoints=1
  To Workspace6 : ToWorkspace  VariableName=L_muscle_states  SampleTime=ts_data
      settings: MaxDataPoints=Inf
  To Workspace7 : ToWorkspace  VariableName=R_muscle_states  SampleTime=ts_data
      settings: MaxDataPoints=Inf
  To Workspace8 : ToWorkspace  VariableName=L_phases  SampleTime=ts_data
      settings: MaxDataPoints=Inf
  To Workspace82 : ToWorkspace  VariableName=maxHeightDiff  SampleTime=-1
      settings: MaxDataPoints=1
  To Workspace9 : ToWorkspace  VariableName=st_sw_decision  SampleTime=ts_data
      settings: MaxDataPoints=Inf
  alpha targets : Subsystem
  track yaw : Subsystem
  wires:
  [numSteps] -> To Workspace3/1
  [stepLengthHist] -> To Workspace4/1
  Clock/1 -> To Workspace28/1
  [fallFlags] -> To Workspace5/1
  [xTorso] -> To Workspace21/1
  Constant1/1 -> To Workspace82/1
  [Lalpha] -> Mux6/2
  [Lalpha_tgt] -> Mux6/3
  [Ralpha] -> Mux6/4
  [Ralpha_tgt] -> Mux6/5
  [Lphi12] -> Mux6/9
  [Lphi23] -> Mux6/8
  [Rphi12] -> Mux6/11
  [Rphi23] -> Mux6/10
  [theta] -> Mux6/1
  Mux7/1 -> To Current Workspace5/1
  "Segment Kinematics (position, orientation)"/1(98) -> Mux7/1  "1:98"
  [xyzTorso] -> Selector1/1
  Selector1/1 -> track yaw/1(xz)
  track yaw/1(yaw) -> Mux7/2  "99"
  [q13] -> Mux/13
  [q11] -> Mux/11
  [q12] -> Mux/12
  [q10] -> Mux/10
  [q9] -> Mux/9
  [q8] -> Mux/8
  [q7] -> Mux/7
  [q6] -> Mux/6
  [q5] -> Mux/5
  [q4] -> Mux/4
  [q3] -> Mux/3
  [q2] -> Mux/2
  [q1] -> Mux/1
  Mux/1 -> To Current Workspace1/1
  [LLength] -> Mux6/6
  [RLength] -> Mux6/7
  [success] -> To Workspace15/1
  Constant2/1 -> To Workspace18/1
  Constant3/1 -> To Workspace19/1
  [Lthigh_cmd_trq] -> Mux3/4
  [Lshin_cmd_trq] -> Mux3/3
  [Rthigh_cmd_trq] -> Mux3/2
  [Rshin_cmd_trq] -> Mux3/1
  [Lthigh_ctrl_trq] -> Mux1/4
  [Lshin_ctrl_trq] -> Mux1/3
  [Rthigh_ctrl_trq] -> Mux1/2
  [Rshin_ctrl_trq] -> Mux1/1
  Mux2/1 -> To Workspace20/1
  Contact and GRFs/1(10) -> Mux7/3  "100:109"
  alpha targets/1(2) -> Mux7/4  "110:111"
  Mux1/1 -> Mux2/1  "desired SEA  torques 1:4"
  Mux3/1 -> Mux2/3  "commanded motor torques 9:12"
  [RM12] -> Mux4/1
  [RM23] -> Mux4/2
  [LM12] -> Mux4/3
  [LM23] -> Mux4/4
  Mux4/1 -> Mux2/4  "desired hip/knee torques 13:16"
  [RM12_sea] -> Mux5/1
  [RM23_sea] -> Mux5/2
  [LM12_sea] -> Mux5/3
  [LM23_sea] -> Mux5/4
  Mux5/1 -> Mux2/5  "commanded hip/knee torques 17:20"
  Mux6/1 -> To Current Workspace2/1
  [LLceHFL] -> Mux19/3  "lce [lopt]"
  [LFmHFL] -> Mux19/2  "F_mtu"
  [LStimHFL] -> Mux19/5  "STIM"
  [LVceHFL] -> Mux19/4  "vce [lopt]"
  [LActHFL] -> Mux19/6  "ACT"
  [LrHFL] -> Mux19/7  "moment arm"
  [LLceGLU] -> Mux18/3  "lce [lopt]"
  [LFmGLU] -> Mux18/2  "F_mtu"
  [LStimGLU] -> Mux18/5  "STIM"
  [LVceGLU] -> Mux18/4  "vce [lopt]"
  [LActGLU] -> Mux18/6  "ACT"
  [LrGLU] -> Mux18/7  "moment arm"
  [LLceHAM] -> Mux20/3  "lce [lopt]"
  [LFmHAM] -> Mux20/2  "F_mtu"
  [LStimHAM] -> Mux20/5  "STIM"
  [LVceHAM] -> Mux20/4  "vce [lopt]"
  [LActHAM] -> Mux20/6  "ACT"
  [LrHAMh] -> Mux20/7  "rh"
  [LrHAMk] -> Mux20/8  "rk"
  [LLceRF] -> Mux21/3  "lce [lopt]"
  [LFmRF] -> Mux21/2  "F_mtu"
  [LStimRF] -> Mux21/5  "STIM"
  [LVceRF] -> Mux21/4  "vce [lopt]"
  [LActRF] -> Mux21/6  "ACT"
  [LrRFh] -> Mux21/7  "rh"
  [LrRFk] -> Mux21/8  "rk"
  [LLceVAS] -> Mux17/3  "lce [lopt]"
  [LFmVAS] -> Mux17/2  "F_mtu"
  [LStimVAS] -> Mux17/5  "STIM"
  [LVceVAS] -> Mux17/4  "vce [lopt]"
  [LActVAS] -> Mux17/6  "ACT"
  [LrVAS] -> Mux17/7  "r"
  [LLceBFSH] -> Mux16/3  "lce [lopt]"
  [LFmBFSH] -> Mux16/2  "F_mtu"
  [LStimBFSH] -> Mux16/5  "STIM"
  [LVceBFSH] -> Mux16/4  "vce [lopt]"
  [LActBFSH] -> Mux16/6  "ACT"
  [LrBFSH] -> Mux16/7  "r"
  Mux20/1 -> Mux12/3  "HAM 15:22"
  Mux18/1 -> Mux12/2  "GLU 8:14"
  Mux19/1 -> Mux12/1  "HFL 1:7"
  Mux21/1 -> Mux12/4  "RF 23:30"
  Mux17/1 -> Mux12/5  "VAS 31:37"
  Mux16/1 -> Mux12/6  "BFSH 38:44"
  Mux12/1 -> To Workspace6/1
  [LLmtuHFL] -> Mux19/1  "L_mtu"
  [LLmtuGLU] -> Mux18/1  "L_mtu"
  [LLmtuHAM] -> Mux20/1  "L_mtu"
  [LLmtuRF] -> Mux21/1  "L_mtu"
  [LLmtuVAS] -> Mux17/1  "L_mtu"
  [LLmtuBFSH] -> Mux16/1  "L_mtu"
  [RLceHFL] -> Mux13/3  "lce [lopt]"
  [RFmHFL] -> Mux13/2  "F_mtu"
  [RStimHFL] -> Mux13/5  "STIM"
  [RVceHFL] -> Mux13/4  "vce [lopt]"
  [RActHFL] -> Mux13/6  "ACT"
  [RrHFL] -> Mux13/7  "moment arm"
  [RLceGLU] -> Mux11/3  "lce [lopt]"
  [RFmGLU] -> Mux11/2  "F_mtu"
  [RStimGLU] -> Mux11/5  "STIM"
  [RVceGLU] -> Mux11/4  "vce [lopt]"
  [RActGLU] -> Mux11/6  "ACT"
  [RrGLU] -> Mux11/7  "moment arm"
  [RLceHAM] -> Mux14/3  "lce [lopt]"
  [RFmHAM] -> Mux14/2  "F_mtu"
  [RStimHAM] -> Mux14/5  "STIM"
  [RVceHAM] -> Mux14/4  "vce [lopt]"
  [RActHAM] -> Mux14/6  "ACT"
  [RrHAMh] -> Mux14/7  "rh"
  [RrHAMk] -> Mux14/8  "rk"
  [RLceRF] -> Mux15/3  "lce [lopt]"
  [RFmRF] -> Mux15/2  "F_mtu"
  [RStimRF] -> Mux15/5  "STIM"
  [RVceRF] -> Mux15/4  "vce [lopt]"
  [RActRF] -> Mux15/6  "ACT"
  [RrRFh] -> Mux15/7  "rh"
  [RrRFk] -> Mux15/8  "rk"
  [RLceVAS] -> Mux10/3  "lce [lopt]"
  [RFmVAS] -> Mux10/2  "F_mtu"
  [RStimVAS] -> Mux10/5  "STIM"
  [RVceVAS] -> Mux10/4  "vce [lopt]"
  [RActVAS] -> Mux10/6  "ACT"
  [RrVAS] -> Mux10/7  "r"
  [RLceBFSH] -> Mux9/3  "lce [lopt]"
  [RFmBFSH] -> Mux9/2  "F_mtu"
  [RStimBFSH] -> Mux9/5  "STIM"
  [RVceBFSH] -> Mux9/4  "vce [lopt]"
  [RActBFSH] -> Mux9/6  "ACT"
  [RrBFSH] -> Mux9/7  "r"
  Mux14/1 -> Mux8/3  "HAM 15:22"
  Mux11/1 -> Mux8/2  "GLU 8:14"
  Mux13/1 -> Mux8/1  "HFL 1:7"
  Mux15/1 -> Mux8/4  "RF 23:30"
  Mux10/1 -> Mux8/5  "VAS 31:37"
  Mux9/1 -> Mux8/6  "BFSH 38:44"
  Mux8/1 -> To Workspace7/1
  [RLmtuHFL] -> Mux13/1  "L_mtu"
  [RLmtuGLU] -> Mux11/1  "L_mtu"
  [RLmtuHAM] -> Mux14/1  "L_mtu"
  [RLmtuRF] -> Mux15/1  "L_mtu"
  [RLmtuVAS] -> Mux10/1  "L_mtu"
  [RLmtuBFSH] -> Mux9/1  "L_mtu"
  Mux22/1 -> Mux2/6  "virtual hip/knee limit torques 21:24"
  [RKneeStop] -> Mux22/1
  [RHipStop] -> Mux22/2
  [LKneeStop] -> Mux22/3
  [LHipStop] -> Mux22/4
  [LtauF] -> Mux23/4
  [LtauB] -> Mux23/3
  [RtauF] -> Mux23/2
  [RtauB] -> Mux23/1
  Mux23/1 -> Mux2/2  "measured SEA  torques 5:8"
  [RLLoad] -> Mux24/1
  [LLLoad] -> Mux24/2
  Mux24/1 -> Mux2/7  "Est. Leg Load 25:26"
  [theta0] -> Mux26/1
  [FPCtrlPar] -> Mux26/2
  [LLCtrlPar] -> Mux26/3
  [StCtrlPar] -> Mux26/4
  [SwCtrlPar] -> Mux26/5
  [TrCtrlPar] -> Mux26/6
  Mux26/1 -> To Workspace1/1
  [RStance] -> Mux27/1  "1"
  [RSwingPhase] -> Mux27/2  "M7-M10 2:5"
  [LStance] -> Mux28/1  "1"
  [LSwingPhase] -> Mux28/2  "M7-M10 2:5"
  [RonL] -> Data Type Conversion/1
  [LonR] -> Data Type Conversion1/1
  [flight] -> Data Type Conversion2/1
  Mux27/1 -> To Workspace2/1
  Mux28/1 -> To Workspace8/1
  Mux29/1 -> To Workspace9/1
  [double_support] -> Data Type Conversion3/1
  [load_footstrike] -> Mux29/5
  [RAct] -> To Workspace10/1
  [LAct] -> To Workspace11/1
  Data Type Conversion/1 -> Mux29/1
  Data Type Conversion1/1 -> Mux29/2
  Data Type Conversion2/1 -> Mux29/3
  Data Type Conversion3/1 -> Mux29/4
  [height_footstrike] -> Mux29/6
  [q] -> To Current Workspace3/1
  [dq] -> To Current Workspace4/1
  [x_com] -> Mux25/1
  [y_com] -> Mux25/2
  [theta] -> Mux25/3
  [dx_com] -> Mux25/4
  [dy_com] -> Mux25/5
  [dtheta] -> Mux25/6
  Mux25/1 -> To Current Workspace7/1
  [NMM_turned_on] -> To Current Workspace6/1

== system ATRIAS_vnmc/control/Import Control Parameters ==
  Constant10 : Constant  Value=TrCtrlPar
  Constant12 : Constant  Value=CtrlPar_theta0
  Constant2 : Constant  Value=LLCtrlPar
  Constant5 : Constant  Value=StCtrlPar
  Constant6 : Constant  Value=FPCtrlPar
  Constant9 : Constant  Value=SwCtrlPar
  tag scope: FPCtrlPar=global, LLCtrlPar=global, StCtrlPar=global, SwCtrlPar=global, TrCtrlPar=global, theta0=global
  wires:
  Constant6/1 -> [FPCtrlPar]
  Constant10/1 -> [TrCtrlPar]
  Constant9/1 -> [SwCtrlPar]
  Constant2/1 -> [LLCtrlPar]
  Constant5/1 -> [StCtrlPar]
  Constant12/1 -> [theta0]

== system ATRIAS_vnmc/control/Lateral Motor Control ==
  note: PD + Buckling Compensation
  Constant : Constant
  Lateral Control1 : MATLAB Function  TreatAsAtomicUnit=on
  Left Lateral Torque Saturation : Saturate  UpperLimit=max_torque_lateral  LowerLimit=-max_torque_lateral
      settings: AttributesFormatString=Top: %<UpperLimit>\nBottom: %<LowerLimit>
  Right Lateral Torque Saturation : Saturate  UpperLimit=max_torque_lateral  LowerLimit=-max_torque_lateral
      settings: AttributesFormatString=Top: %<UpperLimit>\nBottom: %<LowerLimit>
  percent body weight : Gain  Gain=(m_total*g)
  percent body weight1 : Gain  Gain=(m_total*g)
  tau_lateral_R : Outport
  tau_lateral_L : Outport  Port=2
  wires:
  Lateral Control1/1(tau_r) -> Right Lateral Torque Saturation/1
  Lateral Control1/2(tau_l) -> Left Lateral Torque Saturation/1
  Right Lateral Torque Saturation/1 -> tau_lateral_R/1
  Left Lateral Torque Saturation/1 -> tau_lateral_L/1
  [Rphi_Lat] -> Lateral Control1/2(qLateralR)
  [Rdphi_Lat] -> Lateral Control1/3(dqLateralR)
  [Lphi_Lat] -> Lateral Control1/4(qLateralL)
  [Ldphi_Lat] -> Lateral Control1/5(dqLateralL)
  [RLLoad] -> percent body weight/1
  [LLLoad] -> percent body weight1/1
  percent body weight/1 -> Lateral Control1/6(F_leg_R)
  percent body weight1/1 -> Lateral Control1/7(F_leg_L)
  Constant/1 -> Lateral Control1/1(winch_unloaded)
